simulink model "realTimeProcessing"  (R2014a)
settings: Solver=ode45  StartTime=0.0  StopTime=30  RelTol=1e-3
undefined symbols (not defined in the file): numSamplesPer20msFrame
libraries: dspsigops x3, dspxfrm3 x2, dspsrcs4 x1, dspsnks4 x1
settings Model: Creator=Abhi  LastModifiedBy=Abhi
settings DebuggingCC: SolverPrmCheckMsg=none

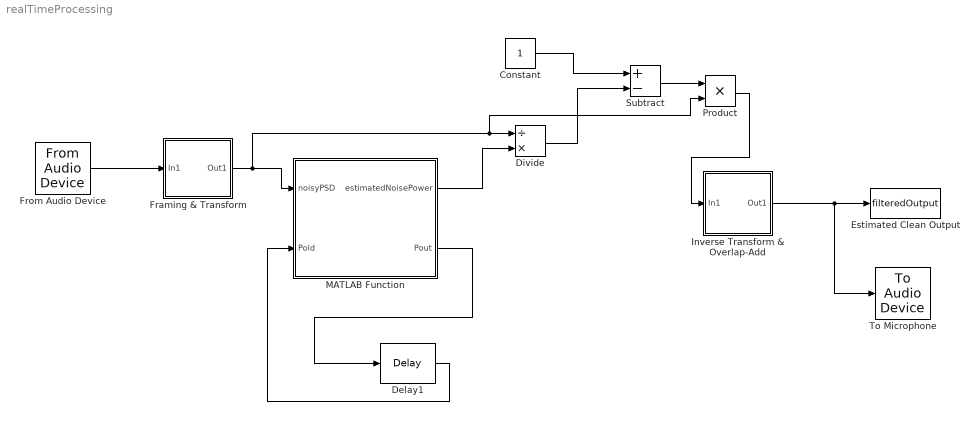
== system realTimeProcessing ==
  Constant : Constant
  Delay1 : dspsigops/Delay  InputProcessing=Columns as channels (frame based)  dly_unit=Frames  delay=1  ic_detail=off  dif_ic_for_ch=off  dif_ic_for_dly=off  ic=0  reset_popup=None
  Divide : Product  Inputs=/*
  Estimated Clean Output : ToWorkspace  VariableName=filteredOutput  SaveFormat=Structure  SampleTime=-1
      settings: Save2DSignal=2-D array (concatenate along first dimension)
  Framing & Transform : Subsystem
  From Audio Device : dspsrcs4/From Audio Device  deviceName=Default  numChannels=1  sampleRate=FS  deviceDatatype=Determine from output data type  autoBufferSize=on  bufferSize=4096  queueDuration=1.0  frameSize=numSamplesPer20msFrame  outputDatatype=double  defaultInputChannelMapping=on  inputChannelMapping=1:2
  Inverse Transform & Overlap-Add : Subsystem
  MATLAB Function : MATLAB Function  TreatAsAtomicUnit=on
  Product : Product
  Subtract : Sum  Inputs=+-
  To Microphone : dspsnks4/To Audio Device  deviceName=Default  inheritSampleRate=on  sampleRate=44100  deviceDatatype=Determine from input data type  autoBufferSize=on  bufferSize=4096  queueDuration=1.0  defaultOutputChannelMapping=on  outputChannelMapping=1:2
  wires:
  From Audio Device/1 -> Framing & Transform/1(In1)
  Inverse Transform & Overlap-Add/1(Out1) -> To Microphone/1, Estimated Clean Output/1
  Framing & Transform/1(Out1) -> Product/2, Divide/1, MATLAB Function/1(noisyPSD)
  MATLAB Function/2(Pout) -> Delay1/1
  Delay1/1 -> MATLAB Function/2(Pold)
  MATLAB Function/1(estimatedNoisePower) -> Divide/2
  Constant/1 -> Subtract/1
  Divide/1 -> Subtract/2
  Subtract/1 -> Product/1
  Product/1 -> Inverse Transform & Overlap-Add/1(In1)

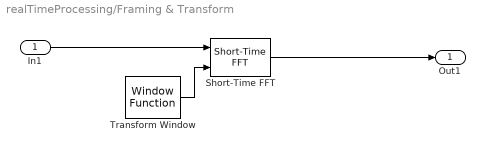
== system realTimeProcessing/Framing & Transform ==
  In1 : Inport
  Short-Time FFT : dspxfrm3/Short-Time FFT  W=numSamplesPer20msFrame  OvLap=overlapSamples  M=numSamplesPer20msFrame  TreatMby1Signals=One channel
  Transform Window : dspsigops/Window Function  winmode=Generate window  wintype=Hanning  sampmode=Discrete  samptime=1  N=numSamplesPer20msFrame  Rs=50  beta=10  winsamp=Symmetric  UserWindow=hamming  OptParams=off  UserParams={'symmetric'}  RowConvenienceOn=on  dataType=double  isSigned=on  wordLen=16  udDataType=sfix(16)  fracBitsMode=Best precision  numFracBits=15  roundingMode=Floor  overflowMode=off  numSidelobes=4  sidelobeLevel=-30
  Out1 : Outport
  wires:
  Short-Time FFT/1 -> Out1/1
  Transform Window/1 -> Short-Time FFT/2
  In1/1 -> Short-Time FFT/1

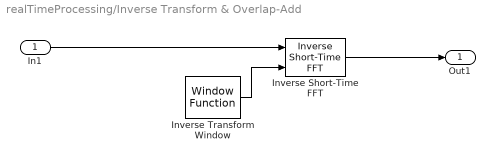
== system realTimeProcessing/Inverse Transform & Overlap-Add ==
  In1 : Inport
  Inverse Transform Window : dspsigops/Window Function  winmode=Generate window  wintype=Hanning  sampmode=Discrete  samptime=1  N=numSamplesPer20msFrame  Rs=50  beta=10  winsamp=Symmetric  UserWindow=hamming  OptParams=off  UserParams={'symmetric'}  RowConvenienceOn=on  dataType=double  isSigned=on  wordLen=16  udDataType=sfix(16)  fracBitsMode=Best precision  numFracBits=15  roundingMode=Floor  overflowMode=off  numSidelobes=4  sidelobeLevel=-30
  Inverse Short-Time FFT : dspxfrm3/Inverse  Short-Time FFT  W=numSamplesPer20msFrame  OvLap=overlapSamples  OutFrameSize=numSamplesPer20msFrame  InConjSymm=on  DoAssert=off  Tol=1e-4
  Out1 : Outport
  wires:
  Inverse Short-Time FFT/1 -> Out1/1
  Inverse Transform Window/1 -> Inverse Short-Time FFT/2
  In1/1 -> Inverse Short-Time FFT/1

== matlab function realTimeProcessing/MATLAB Function ==
  data: noisyPSD input; estimatedNoisePower output; Pold input; Pout output
function [estimatedNoisePower, Pout]  = estNoisePowerMS(noisyPSD, Pold)

    alpha = 0.9999;
    
    P = alpha*Pold + (1-alpha)*noisyPSD;
    
    estimatedNoisePower = real(min(P, Pold)./((P+Pold)/2));
    Pout = real(P);    
end
